simulink model "lift_drag"  (R2024a)
settings: Solver=VariableStepAuto  StartTime=0.0  StopTime=10.0  RelTol=1e-3
InitFcn:
  | %% CONFIGURATION GOEMETRY MODELLING
  | 
  | fuse_dia = 0.3; % m
  | braket_space = 0.05; % m
  | num_ab = 3;
  | ab_span = 0.9; % m
  | ab_chord = 0.6844; % m
  | sys_CG = -0.6; % m; respect to top of fuselage
  | 
  | 
  | ab_cd = 2.2;
  | cyl_cd = 0.8;
settings Model: Creator=thoma  LastModifiedBy=thoma

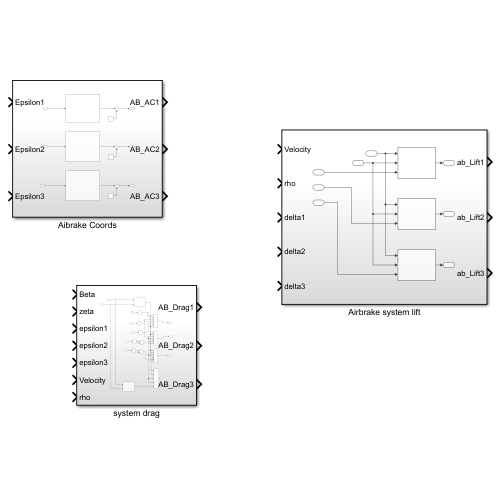
[thumbnail: Simulink's stored preview of the top-level diagram]
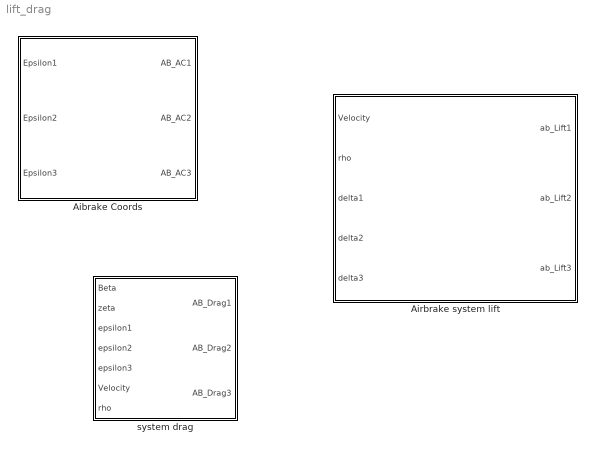
== system lift_drag ==
  Aibrake Coords : Subsystem
  Airbrake system lift : Subsystem
  system drag : Subsystem

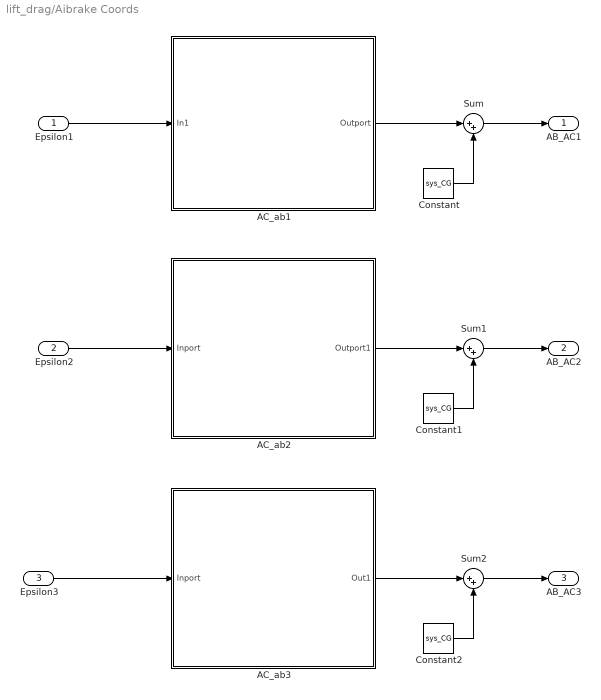
== system lift_drag/Aibrake Coords ==
  Epsilon1 : Inport
  Epsilon2 : Inport  Port=2
  Epsilon3 : Inport  Port=3
  AC_ab1 : Subsystem
  AC_ab2 : Subsystem
  AC_ab3 : Subsystem
  Constant : Constant  Value=sys_CG
  Constant1 : Constant  Value=sys_CG
  Constant2 : Constant  Value=sys_CG
  Sum : Sum  Inputs=|++
  Sum1 : Sum  Inputs=|++
  Sum2 : Sum  Inputs=|++
  AB_AC1 : Outport
  AB_AC2 : Outport  Port=2
  AB_AC3 : Outport  Port=3
  wires:
  Epsilon1/1 -> AC_ab1/1(In1)
  Epsilon2/1 -> AC_ab2/1(Inport)
  Epsilon3/1 -> AC_ab3/1(Inport)
  AC_ab1/1(Outport) -> Sum/1
  Constant/1 -> Sum/2
  Sum/1 -> AB_AC1/1
  Constant1/1 -> Sum1/2
  Sum1/1 -> AB_AC2/1
  AC_ab2/1(Outport1) -> Sum1/1
  Constant2/1 -> Sum2/2
  Sum2/1 -> AB_AC3/1
  AC_ab3/1(Out1) -> Sum2/1

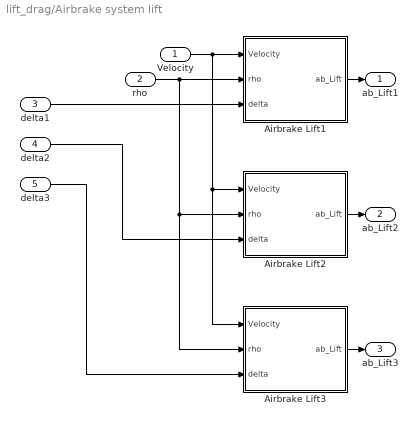
== system lift_drag/Airbrake system lift ==
  Velocity : Inport
  rho : Inport  Port=2
  delta1 : Inport  Port=3
  delta2 : Inport  Port=4
  delta3 : Inport  Port=5
  Airbrake Lift1 : Subsystem
  Airbrake Lift2 : Subsystem
  Airbrake Lift3 : Subsystem
  ab_Lift1 : Outport
  ab_Lift2 : Outport  Port=2
  ab_Lift3 : Outport  Port=3
  wires:
  Airbrake Lift1/1(ab_Lift) -> ab_Lift1/1
  Velocity/1 -> Airbrake Lift3/1(Velocity), Airbrake Lift2/1(Velocity), Airbrake Lift1/1(Velocity)
  rho/1 -> Airbrake Lift3/2(rho), Airbrake Lift2/2(rho), Airbrake Lift1/2(rho)
  delta1/1 -> Airbrake Lift1/3(delta)
  delta2/1 -> Airbrake Lift2/3(delta)
  Airbrake Lift2/1(ab_Lift) -> ab_Lift2/1
  delta3/1 -> Airbrake Lift3/3(delta)
  Airbrake Lift3/1(ab_Lift) -> ab_Lift3/1

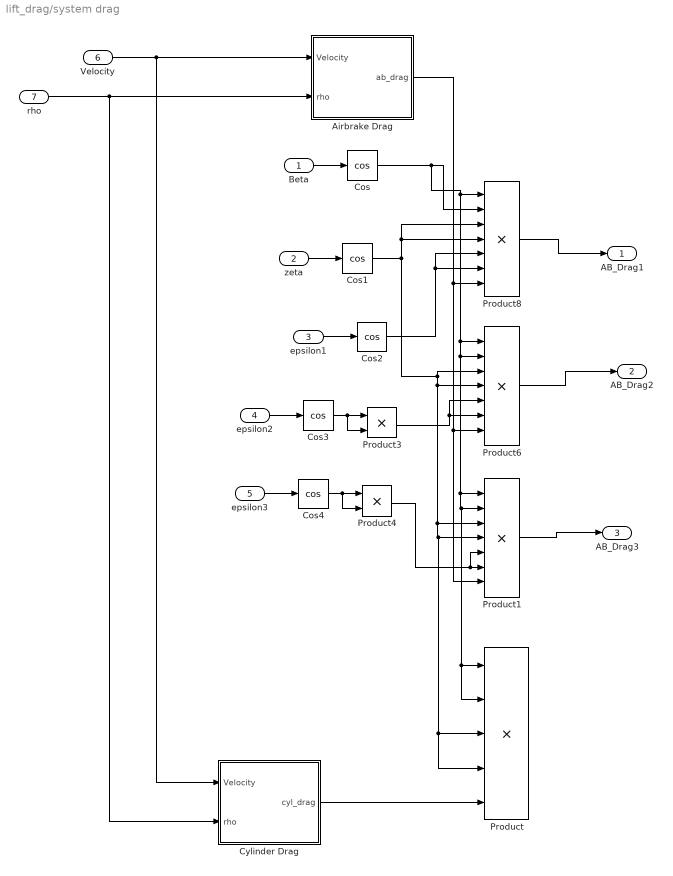
== system lift_drag/system drag ==
  Beta : Inport
  zeta : Inport  Port=2
  epsilon1 : Inport  Port=3
  epsilon2 : Inport  Port=4
  epsilon3 : Inport  Port=5
  Velocity : Inport  Port=6
  rho : Inport  Port=7
  Airbrake Drag : Subsystem
  Cos{,1..4} (5 alike) : Trigonometry  Operator=cos
  Cylinder Drag : Subsystem
  Product : Product  Inputs=5
  Product1 : Product  Inputs=7
  Product3 : Product
  Product4 : Product
  Product6 : Product  Inputs=7
  Product8 : Product  Inputs=7
  AB_Drag1 : Outport
  AB_Drag2 : Outport  Port=2
  AB_Drag3 : Outport  Port=3
  wires:
  Cos/1 -> Product8/2, Product/2, Product/1, Product1/2, Product1/1, Product6/2, Product6/1, Product8/1
  Beta/1 -> Cos/1
  Cos1/1 -> Product8/4, Product8/3, Product/4, Product/3, Product1/4, Product1/3, Product6/4, Product6/3
  zeta/1 -> Cos1/1
  Cos2/1 -> Product8/6, Product8/5
  epsilon1/1 -> Cos2/1
  Cos3/1 -> Product3/2, Product3/1
  epsilon2/1 -> Cos3/1
  Cos4/1 -> Product4/2, Product4/1
  epsilon3/1 -> Cos4/1
  Product3/1 -> Product6/6, Product6/5
  Product4/1 -> Product1/6, Product1/5
  Product8/1 -> AB_Drag1/1
  Product6/1 -> AB_Drag2/1
  Product1/1 -> AB_Drag3/1
  Airbrake Drag/1(ab_drag) -> Product1/7, Product6/7, Product8/7
  Velocity/1 -> Cylinder Drag/1(Velocity), Airbrake Drag/1(Velocity)
  rho/1 -> Cylinder Drag/2(rho), Airbrake Drag/2(rho)
  Cylinder Drag/1(cyl_drag) -> Product/5

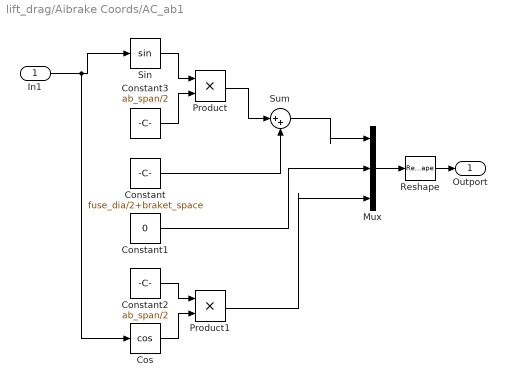
== system lift_drag/Aibrake Coords/AC_ab1 ==
  In1 : Inport
  Constant : Constant  Value=fuse_dia/2+braket_space
  Constant1 : Constant  Value=0
  Constant2 : Constant  Value=ab_span/2
  Constant3 : Constant  Value=ab_span/2
  Cos : Trigonometry  Operator=cos
  Mux : Mux  Inputs=3
  Product : Product
  Product1 : Product
  Reshape : Reshape  OutputDimensionality=Row vector (2-D)
  Sin : Trigonometry
  Sum : Sum  Inputs=|++
  Outport : Outport
  wires:
  Cos/1 -> Product1/2
  Mux/1 -> Reshape/1
  Constant/1 -> Sum/2
  In1/1 -> Cos/1, Sin/1
  Constant1/1 -> Mux/2
  Sin/1 -> Product/1
  Constant2/1 -> Product1/1
  Product/1 -> Sum/1
  Constant3/1 -> Product/2
  Product1/1 -> Mux/3
  Sum/1 -> Mux/1
  Reshape/1 -> Outport/1

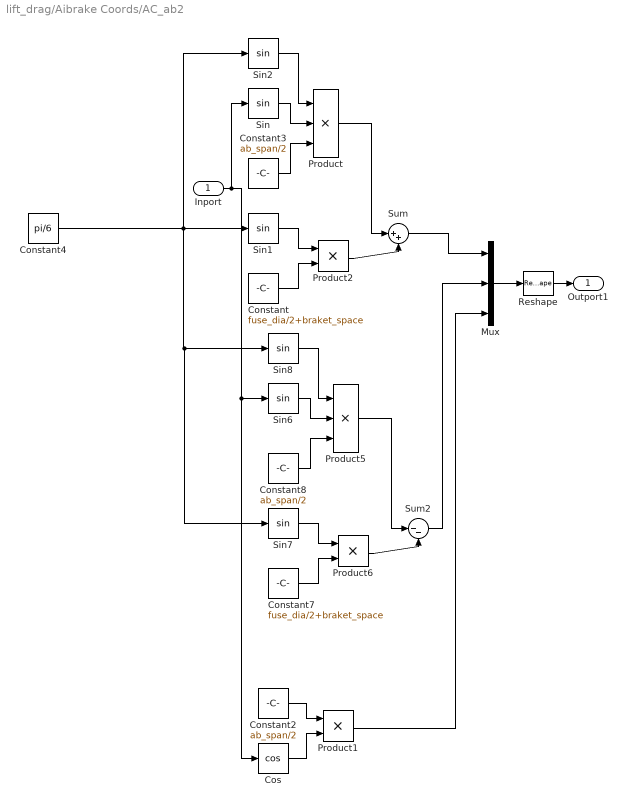
== system lift_drag/Aibrake Coords/AC_ab2 ==
  Inport : Inport
  Constant : Constant  Value=fuse_dia/2+braket_space
  Constant2 : Constant  Value=ab_span/2
  Constant3 : Constant  Value=ab_span/2
  Constant4 : Constant  Value=pi/6
  Constant7 : Constant  Value=fuse_dia/2+braket_space
  Constant8 : Constant  Value=ab_span/2
  Cos : Trigonometry  Operator=cos
  Mux : Mux  Inputs=3
  Product : Product  Inputs=3
  Product1 : Product
  Product2 : Product
  Product5 : Product  Inputs=3
  Product6 : Product
  Reshape : Reshape  OutputDimensionality=Row vector (2-D)
  Sin{,1..2,6..8} (6 alike) : Trigonometry
  Sum : Sum  Inputs=|++
  Sum2 : Sum  Inputs=|--
  Outport1 : Outport
  wires:
  Cos/1 -> Product1/2
  Mux/1 -> Reshape/1
  Inport/1 -> Sin6/1, Cos/1, Sin/1
  Constant2/1 -> Product1/1
  Product/1 -> Sum/1
  Product1/1 -> Mux/3
  Sum/1 -> Mux/1
  Reshape/1 -> Outport1/1
  Sin1/1 -> Product2/1
  Constant/1 -> Product2/2
  Product2/1 -> Sum/2
  Constant3/1 -> Product/3
  Sin/1 -> Product/2
  Sin2/1 -> Product/1
  Constant4/1 -> Sin7/1, Sin8/1, Sin2/1, Sin1/1
  Sin6/1 -> Product5/2
  Constant8/1 -> Product5/3
  Sin7/1 -> Product6/1
  Sin8/1 -> Product5/1
  Product5/1 -> Sum2/1
  Product6/1 -> Sum2/2
  Constant7/1 -> Product6/2
  Sum2/1 -> Mux/2

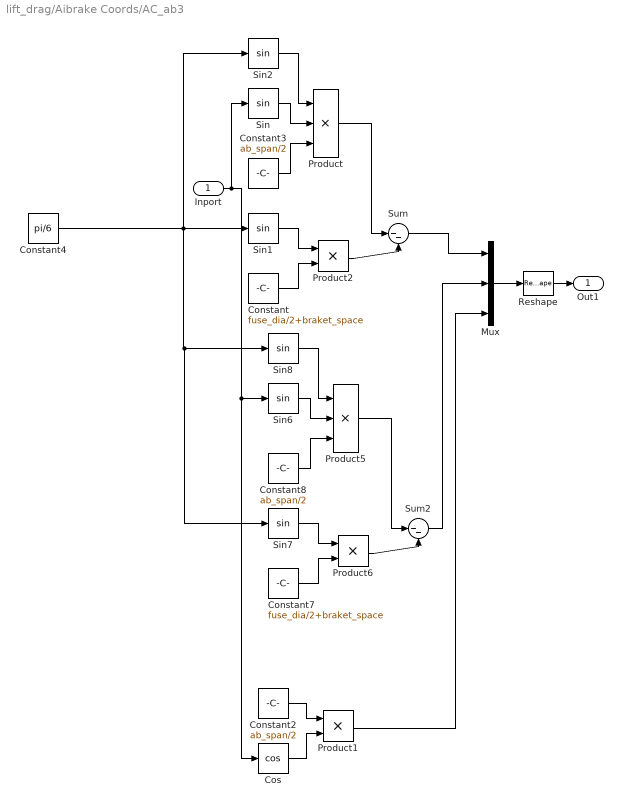
== system lift_drag/Aibrake Coords/AC_ab3 ==
  Inport : Inport
  Constant : Constant  Value=fuse_dia/2+braket_space
  Constant2 : Constant  Value=ab_span/2
  Constant3 : Constant  Value=ab_span/2
  Constant4 : Constant  Value=pi/6
  Constant7 : Constant  Value=fuse_dia/2+braket_space
  Constant8 : Constant  Value=ab_span/2
  Cos : Trigonometry  Operator=cos
  Mux : Mux  Inputs=3
  Product : Product  Inputs=3
  Product1 : Product
  Product2 : Product
  Product5 : Product  Inputs=3
  Product6 : Product
  Reshape : Reshape  OutputDimensionality=Row vector (2-D)
  Sin{,1..2,6..8} (6 alike) : Trigonometry
  Sum : Sum  Inputs=|--
  Sum2 : Sum  Inputs=|--
  Out1 : Outport
  wires:
  Cos/1 -> Product1/2
  Mux/1 -> Reshape/1
  Inport/1 -> Sin6/1, Cos/1, Sin/1
  Constant2/1 -> Product1/1
  Product/1 -> Sum/1
  Product1/1 -> Mux/3
  Sum/1 -> Mux/1
  Reshape/1 -> Out1/1
  Sin1/1 -> Product2/1
  Constant/1 -> Product2/2
  Product2/1 -> Sum/2
  Constant3/1 -> Product/3
  Sin/1 -> Product/2
  Sin2/1 -> Product/1
  Constant4/1 -> Sin7/1, Sin8/1, Sin2/1, Sin1/1
  Sin6/1 -> Product5/2
  Constant8/1 -> Product5/3
  Sin7/1 -> Product6/1
  Sin8/1 -> Product5/1
  Product5/1 -> Sum2/1
  Product6/1 -> Sum2/2
  Constant7/1 -> Product6/2
  Sum2/1 -> Mux/2

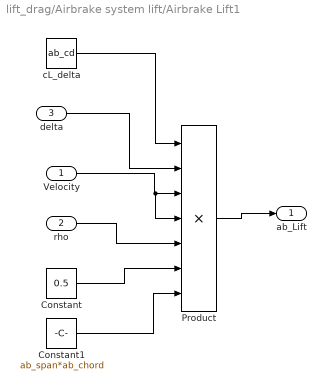
== system lift_drag/Airbrake system lift/Airbrake Lift1 ==
  Velocity : Inport
  rho : Inport  Port=2
  delta : Inport  Port=3
  Constant : Constant  Value=0.5
  Constant1 : Constant  Value=ab_span*ab_chord
  Product : Product  Inputs=7
  cL_delta : Constant  Value=ab_cd
  ab_Lift : Outport
  wires:
  Velocity/1 -> Product/4, Product/3
  Product/1 -> ab_Lift/1
  cL_delta/1 -> Product/1
  delta/1 -> Product/2
  rho/1 -> Product/5
  Constant/1 -> Product/6
  Constant1/1 -> Product/7

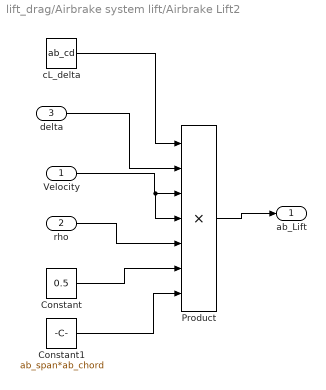
== system lift_drag/Airbrake system lift/Airbrake Lift2 ==
  Velocity : Inport
  rho : Inport  Port=2
  delta : Inport  Port=3
  Constant : Constant  Value=0.5
  Constant1 : Constant  Value=ab_span*ab_chord
  Product : Product  Inputs=7
  cL_delta : Constant  Value=ab_cd
  ab_Lift : Outport
  wires:
  Velocity/1 -> Product/4, Product/3
  Product/1 -> ab_Lift/1
  cL_delta/1 -> Product/1
  delta/1 -> Product/2
  rho/1 -> Product/5
  Constant/1 -> Product/6
  Constant1/1 -> Product/7

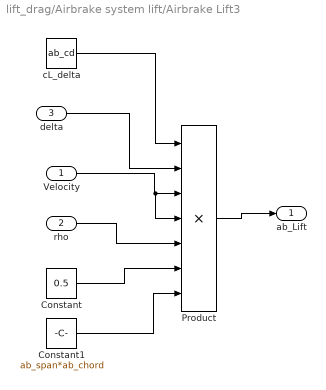
== system lift_drag/Airbrake system lift/Airbrake Lift3 ==
  Velocity : Inport
  rho : Inport  Port=2
  delta : Inport  Port=3
  Constant : Constant  Value=0.5
  Constant1 : Constant  Value=ab_span*ab_chord
  Product : Product  Inputs=7
  cL_delta : Constant  Value=ab_cd
  ab_Lift : Outport
  wires:
  Velocity/1 -> Product/4, Product/3
  Product/1 -> ab_Lift/1
  cL_delta/1 -> Product/1
  delta/1 -> Product/2
  rho/1 -> Product/5
  Constant/1 -> Product/6
  Constant1/1 -> Product/7

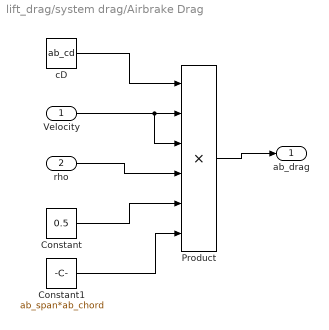
== system lift_drag/system drag/Airbrake Drag ==
  Velocity : Inport
  rho : Inport  Port=2
  Constant : Constant  Value=0.5
  Constant1 : Constant  Value=ab_span*ab_chord
  Product : Product  Inputs=6
  cD : Constant  Value=ab_cd
  ab_drag : Outport
  wires:
  cD/1 -> Product/1
  Velocity/1 -> Product/3, Product/2
  rho/1 -> Product/4
  Constant/1 -> Product/5
  Constant1/1 -> Product/6
  Product/1 -> ab_drag/1

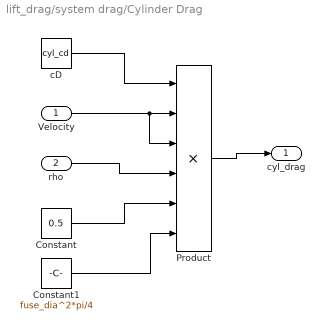
== system lift_drag/system drag/Cylinder Drag ==
  Velocity : Inport
  rho : Inport  Port=2
  Constant : Constant  Value=0.5
  Constant1 : Constant  Value=fuse_dia^2*pi/4
  Product : Product  Inputs=6
  cD : Constant  Value=cyl_cd
  cyl_drag : Outport
  wires:
  cD/1 -> Product/1
  Velocity/1 -> Product/3, Product/2
  rho/1 -> Product/4
  Constant/1 -> Product/5
  Constant1/1 -> Product/6
  Product/1 -> cyl_drag/1
